simulink model "DKM"  (R2015a)
settings: Solver=ode3  StartTime=0.0  StopTime=10.0  FixedStep=0.1  RelTol=1e-3
values from neighbouring files (symbols this model uses):
  L = 0.13    [Init.m]    (also in KinematicPlot.m; plotVehicle.m)
  qdot = [2;0]    [KinematicPlot.m]
  r = 0.1    [Init.m]    (also in KinematicPlot.m)
settings Model: Creator=tgvo  LastModifiedBy=tgvo

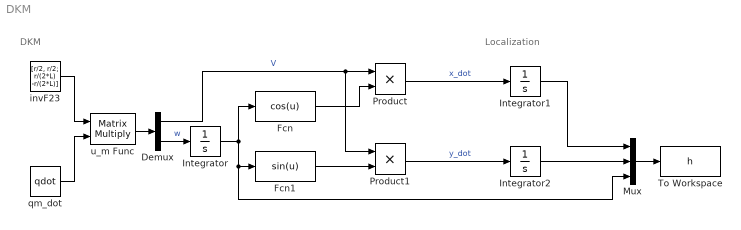
== system DKM ==
  note: DKM
  note: Localization
  Demux : Demux  Outputs=2
  Fcn : Fcn  Expr=cos(u)
  Fcn1 : Fcn  Expr=sin(u)
  Integrator : Integrator
  Integrator1 : Integrator
  Integrator2 : Integrator
  Mux : Mux  Inputs=3
  Product : Product
  Product1 : Product
  To Workspace : ToWorkspace  VariableName=h  SampleTime=-1
  invF23 : Constant  Value=[r/2, r/2; r/(2*L) -r/(2*L)]
  qm_dot : Constant  Value=qdot
  u_m Func : Product  Multiplication=Matrix(*)
  wires:
  Integrator/1 -> Mux/3, Fcn1/1, Fcn/1
  Integrator2/1 -> Mux/2
  Integrator1/1 -> Mux/1
  Mux/1 -> To Workspace/1
  Fcn1/1 -> Product1/2
  Fcn/1 -> Product/2
  Demux/1 -> Product1/1, Product/1  "V"
  Demux/2 -> Integrator/1  "w"
  u_m Func/1 -> Demux/1
  Product1/1 -> Integrator2/1  "y_dot"
  Product/1 -> Integrator1/1  "x_dot"
  invF23/1 -> u_m Func/1
  qm_dot/1 -> u_m Func/2
